simulink model "basicSISOsimulation"  (R2019b)
settings: Solver=VariableStepAuto  StartTime=0.0  StopTime=2  FixedStep=0.05  RelTol=1e-3
PreLoadFcn:
  | loadSystemVariables
values from neighbouring files (symbols this model uses):
  I = qpar('I',0.050,0.040,0.060,50)    [SISO_phi.m]    (also in SISO_x.m = 0.05; basicSISO_phi.m; basicSISO_x.m = 0.05; basicSISO_y.m = 0.05)
  m_nom = 1    [SISO_x.m]    (also in basicSISO_x.m; basicSISO_y.m; loadSystemVariables.m)
  tau = 0.075    [loadSystemVariables.m]
  tau2 = qpar('tau2',0.060,0.050,0.070,50)    [SISO_phi.m]    (also in loadSystemVariables.m = 0.06)
libraries: cstblocks x8, simulink_extras x2, aerolibguid x1, simulink x1
settings Model: Creator=Iftah  LastModifiedBy=Iftah
settings SolverCC: ZeroCrossAlgorithm=Adaptive  AlgebraicLoopSolver=LineSearch
settings DebuggingCC: IgnoredZcDiagnostic=none

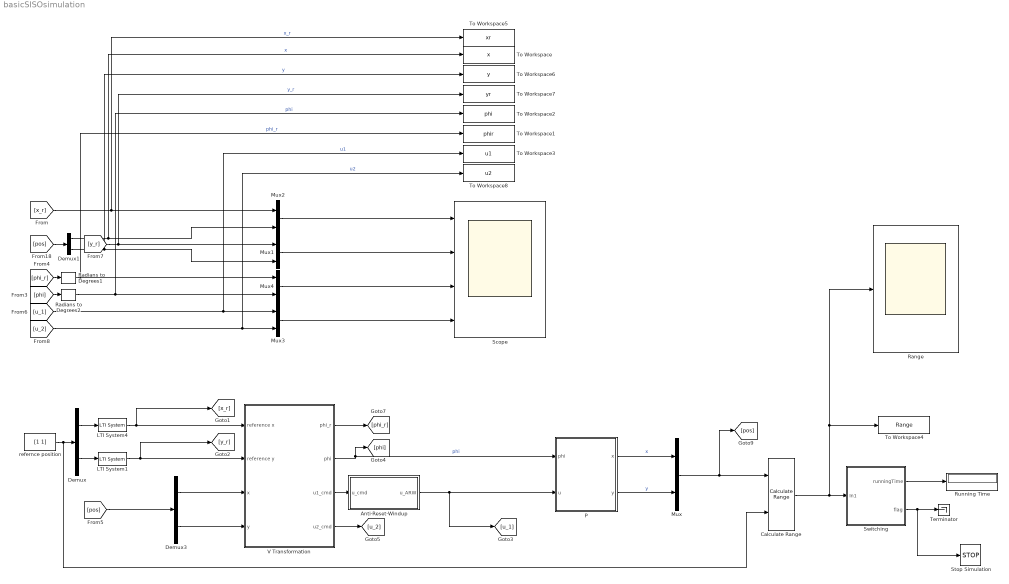
== system basicSISOsimulation ==
  Anti-Reset-Windup : Subsystem
  Calculate Range : aerolibguid/Calculate Range
      settings: SourceProductName=Aerospace Blockset  SourceProductBaseCode=AE
  Demux : Demux  Outputs=2
  Demux1 : Demux  Outputs=2
  Demux3 : Demux  Outputs=2
  LTI System1 : cstblocks/LTI System  sys=Fv  IC=[]
  LTI System4 : cstblocks/LTI System  sys=Fv  IC=[]
  Mux{,1..4} (5 alike) : Mux  Inputs=2
  P : Subsystem
  Radians to Degrees1 : simulink_extras/Transformations/Radians to Degrees
  Radians to Degrees2 : simulink_extras/Transformations/Radians to Degrees
  Range : Scope
  Running Time : Display
  Scope : Scope  NumInputPorts=4
  Stop Simulation : Stop
  Switching : Subsystem
  Terminator : Terminator
  To Workspace : ToWorkspace  VariableName=x  SaveFormat=Timeseries  SampleTime=-1
  To Workspace1 : ToWorkspace  VariableName=phir  SaveFormat=Timeseries  SampleTime=-1
  To Workspace2 : ToWorkspace  VariableName=phi  SaveFormat=Timeseries  SampleTime=-1
  To Workspace3 : ToWorkspace  VariableName=u1  SaveFormat=Timeseries  SampleTime=-1
  To Workspace4 : ToWorkspace  VariableName=Range  SaveFormat=Timeseries  SampleTime=-1
  To Workspace5 : ToWorkspace  VariableName=xr  SaveFormat=Timeseries  SampleTime=-1
  To Workspace6 : ToWorkspace  VariableName=y  SaveFormat=Timeseries  SampleTime=-1
  To Workspace7 : ToWorkspace  VariableName=yr  SaveFormat=Timeseries  SampleTime=-1
  To Workspace8 : ToWorkspace  VariableName=u2  SaveFormat=Timeseries  SampleTime=-1
  V Transformation : Subsystem
  "refernce position " : Constant  Value=[1 1]
  wires:
  "refernce position "/1 -> Demux/1, Calculate Range/2
  Demux/1 -> LTI System4/1
  Demux/2 -> LTI System1/1
  V Transformation/2(phi) -> [phi], P/1(phi)  "phi"
  Mux1/1 -> Scope/2
  Mux2/1 -> Scope/1
  [x_r] -> To Workspace5/1, Mux2/1  "x_r"
  Demux1/1 -> To Workspace/1, Mux2/2  "x"
  Demux1/2 -> Mux1/2, To Workspace6/1  "y"
  [y_r] -> Mux1/1, To Workspace7/1  "y_r"
  Mux4/1 -> Scope/3
  Mux3/1 -> Scope/4
  [u_1] -> To Workspace3/1, Mux3/1  "u1"
  [u_2] -> To Workspace8/1, Mux3/2  "u2"
  V Transformation/1(phi_r) -> [phi_r]
  [phi_r] -> Radians to Degrees1/1
  [phi] -> Radians to Degrees2/1
  Radians to Degrees1/1 -> Mux4/1, To Workspace1/1  "phi_r"
  Radians to Degrees2/1 -> To Workspace2/1, Mux4/2  "phi"
  P/1(x) -> Mux/1  "x"
  P/2(y) -> Mux/2  "y"
  Demux3/1 -> V Transformation/3(x)
  Demux3/2 -> V Transformation/4(y)
  Calculate Range/1 -> Switching/1(In1), To Workspace4/1, Range/1
  Switching/1(runningTime) -> Running Time/1
  LTI System4/1 -> [x_r], V Transformation/1(reference x)
  LTI System1/1 -> [y_r], V Transformation/2(reference y)
  [pos] -> Demux1/1
  V Transformation/4(u2_cmd) -> [u_2]
  Switching/2("flag ") -> Stop Simulation/1, Terminator/1
  Mux/1 -> [pos], Calculate Range/1
  [pos] -> Demux3/1
  V Transformation/3(u1_cmd) -> Anti-Reset-Windup/1(u_cmd)
  Anti-Reset-Windup/1(u_ARW) -> P/2("u "), [u_1]

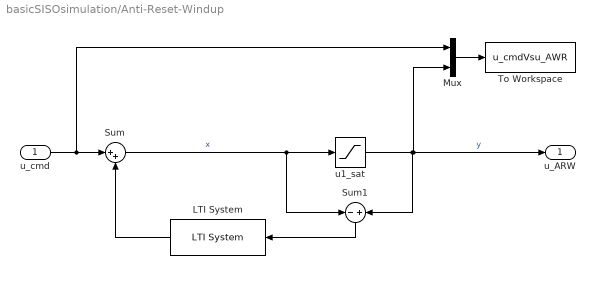
== system basicSISOsimulation/Anti-Reset-Windup ==
  u_cmd : Inport
  LTI System : cstblocks/LTI System  sys=Hv  IC=[]
  Mux : Mux  Inputs=2
  Sum : Sum  Inputs=|++
  Sum1 : Sum  Inputs=-|+
  To Workspace : ToWorkspace  VariableName=u_cmdVsu_AWR  SaveFormat=Timeseries  SampleTime=-1
  u1_sat : Saturate  UpperLimit=25  LowerLimit=-25
  u_ARW : Outport
  wires:
  u_cmd/1 -> Mux/1, Sum/1
  u1_sat/1 -> Mux/2, u_ARW/1, Sum1/2  "y"
  Sum/1 -> Sum1/1, u1_sat/1  "x"
  Sum1/1 -> LTI System/1
  LTI System/1 -> Sum/2
  Mux/1 -> To Workspace/1

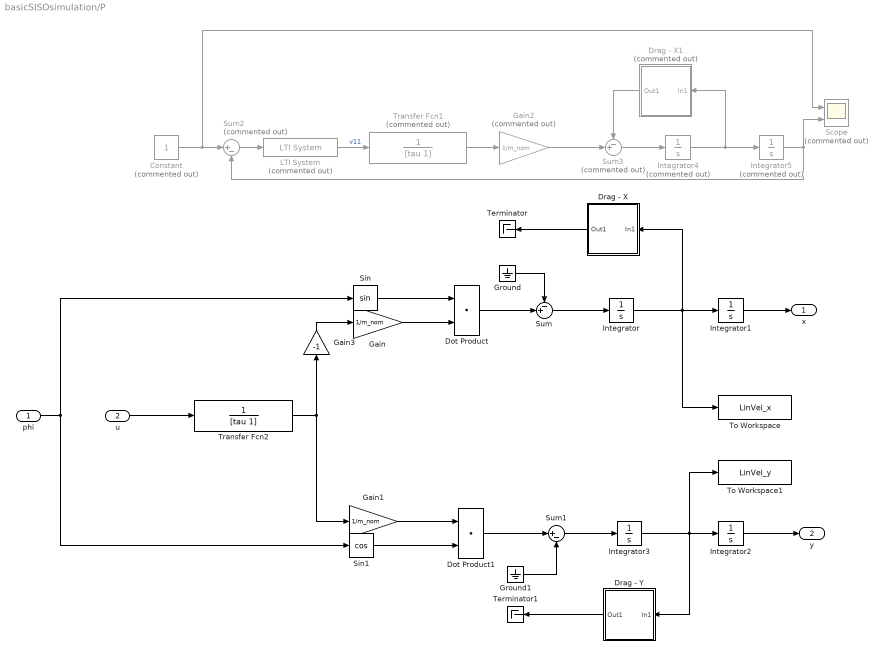
== system basicSISOsimulation/P ==
  phi : Inport
  "u " : Inport  Port=2
  Constant : Constant  Commented=on
  Dot Product : DotProduct  InputSameDT=on  OutDataTypeStr=Inherit: Inherit via internal rule
  Dot Product1 : DotProduct  InputSameDT=on  OutDataTypeStr=Inherit: Inherit via internal rule
  Drag - X : Subsystem
  Drag - X1 : Subsystem  Commented=on
  Drag - Y : Subsystem
  Gain : Gain  Gain=1/m_nom
  Gain1 : Gain  Gain=1/m_nom
  Gain2 : Gain  Commented=on  Gain=1/m_nom
  Gain3 : Gain  Gain=-1
  Ground : Ground
  Ground1 : Ground
  Integrator : Integrator
  Integrator1 : Integrator  InitialCondition=1e-3
  Integrator2 : Integrator  InitialCondition=1e-3
  Integrator3 : Integrator
  Integrator4 : Integrator  Commented=on  InitialCondition=1e-3
  Integrator5 : Integrator  Commented=on  InitialCondition=1e-3
  LTI System : cstblocks/LTI System  Commented=on  sys=Gv  IC=[]
  Scope : Scope  Commented=on  NumInputPorts=2
  Sin : Trigonometry
  Sin1 : Trigonometry  Operator=cos
  Sum : Sum  Inputs=-+|
  Sum1 : Sum  Inputs=|+-
  Sum2 : Sum  Commented=on  Inputs=|+-
  Sum3 : Sum  Commented=on  Inputs=-+|
  Terminator : Terminator
  Terminator1 : Terminator
  To Workspace : ToWorkspace  VariableName=LinVel_x  SaveFormat=Timeseries  SampleTime=-1
  To Workspace1 : ToWorkspace  VariableName=LinVel_y  SaveFormat=Timeseries  SampleTime=-1
  Transfer Fcn1 : TransferFcn  Commented=on  Denominator=[tau 1]
  Transfer Fcn2 : TransferFcn  Denominator=[tau 1]
  x : Outport
  y : Outport  Port=2
  wires:
  Gain/1 -> Dot Product/2
  Integrator1/1 -> x/1
  Integrator3/1 -> Drag - Y/1(In1), To Workspace1/1, Integrator2/1
  phi/1 -> Sin/1, Sin1/1
  Sin1/1 -> Dot Product1/2
  Gain3/1 -> Gain/1
  Gain1/1 -> Dot Product1/1
  "u "/1 -> Transfer Fcn2/1
  Transfer Fcn2/1 -> Gain1/1, Gain3/1
  Sin/1 -> Dot Product/1
  Integrator/1 -> To Workspace/1, Integrator1/1, Drag - X/1(In1)
  Sum/1 -> Integrator/1
  Sum1/1 -> Integrator3/1
  Drag - Y/1(Out1) -> Terminator1/1
  Dot Product/1 -> Sum/2
  Dot Product1/1 -> Sum1/1
  Transfer Fcn1/1 -> Gain2/1
  LTI System/1 -> Transfer Fcn1/1  "v11"
  Sum2/1 -> LTI System/1
  Constant/1 -> Scope/1, Sum2/1
  Integrator2/1 -> y/1
  Integrator4/1 -> Drag - X1/1(In1), Integrator5/1
  Gain2/1 -> Sum3/2
  Integrator5/1 -> Scope/2, Sum2/2
  Sum3/1 -> Integrator4/1
  Drag - X1/1(Out1) -> Sum3/1
  Drag - X/1(Out1) -> Terminator/1
  Ground/1 -> Sum/1
  Ground1/1 -> Sum1/2

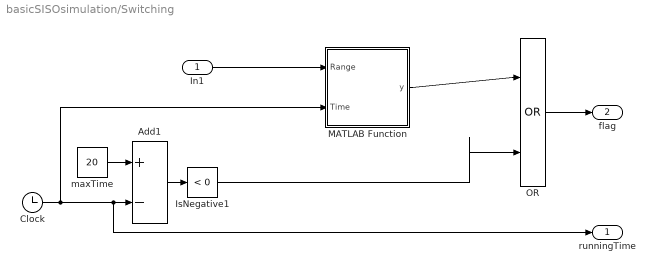
== system basicSISOsimulation/Switching ==
  In1 : Inport
  Add1 : Sum  Inputs=+-
  Clock : Clock
  IsNegative1 : simulink/Logic and Bit Operations/Compare To Zero  relop=<  OutDataTypeStr=boolean
  MATLAB Function : MATLAB Function  TreatAsAtomicUnit=on
  OR : Logic  Operator=OR  IconShape=distinctive  AllPortsSameDT=off  OutDataTypeStr=boolean
  maxTime : Constant  Value=20
  runningTime : Outport
  "flag " : Outport  Port=2
  wires:
  OR/1 -> "flag "/1
  IsNegative1/1 -> OR/2
  Add1/1 -> IsNegative1/1
  In1/1 -> MATLAB Function/1(Range)
  Clock/1 -> MATLAB Function/2(Time), runningTime/1, Add1/2
  maxTime/1 -> Add1/1
  MATLAB Function/1(y) -> OR/1

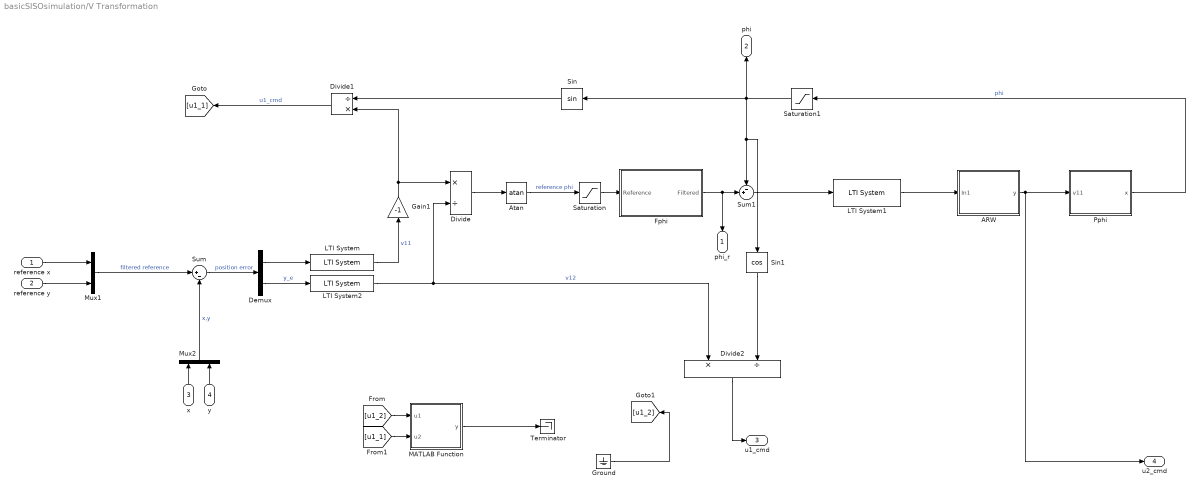
== system basicSISOsimulation/V Transformation ==
  reference x : Inport
  reference y : Inport  Port=2
  x : Inport  Port=3
  y : Inport  Port=4
  ARW : Subsystem
  Atan : Trigonometry  Operator=atan
  Demux : Demux  Outputs=2
  Divide : Product  Inputs=*/
  Divide1 : Product  Inputs=/*
  Divide2 : Product  Inputs=*/
  Fphi : Subsystem
  Gain1 : Gain  Gain=-1
  Ground : Ground
  LTI System : cstblocks/LTI System  sys=Gv  IC=[]
  LTI System1 : cstblocks/LTI System  sys=Gphi  IC=[]
  LTI System2 : cstblocks/LTI System  sys=Gv  IC=[]
  MATLAB Function : MATLAB Function  TreatAsAtomicUnit=on
  Mux1 : Mux  Inputs=2
  Mux2 : Mux  Inputs=2
  Pphi : Subsystem
  Saturation : Saturate  UpperLimit=pi/3  LowerLimit=-pi/3
  Saturation1 : Saturate  UpperLimit=pi/3  LowerLimit=-pi/3
  Sin : Trigonometry
  Sin1 : Trigonometry  Operator=cos
  Sum : Sum  Inputs=|+-
  Sum1 : Sum  Inputs=-+|
  Terminator : Terminator
  phi_r : Outport
  phi : Outport  Port=2
  u1_cmd : Outport  Port=3
  u2_cmd : Outport  Port=4
  wires:
  Divide/1 -> Atan/1
  LTI System2/1 -> Divide2/1, Divide/2  "v12"
  Pphi/1(x) -> Saturation1/1  "phi"
  Sum/1 -> Demux/1  "position error"
  Sum1/1 -> LTI System1/1
  Demux/2 -> LTI System2/1  "y_e"
  Mux1/1 -> Sum/1  "filtered reference"
  Atan/1 -> Saturation/1  "reference phi"
  y/1 -> Mux2/2
  x/1 -> Mux2/1
  Mux2/1 -> Sum/2  "x,y"
  reference y/1 -> Mux1/2
  reference x/1 -> Mux1/1
  Sin1/1 -> Divide2/2
  Gain1/1 -> Divide/1, Divide1/2
  LTI System/1 -> Gain1/1  "v11"
  Divide1/1 -> [u1_1]  "u1_cmd"
  Sin/1 -> Divide1/1
  Divide2/1 -> u1_cmd/1
  Demux/1 -> LTI System/1
  [u1_2] -> MATLAB Function/1(u1)
  [u1_1] -> MATLAB Function/2(u2)
  MATLAB Function/1(y) -> Terminator/1
  Fphi/1(Filtered) -> Sum1/2, phi_r/1
  LTI System1/1 -> ARW/1(In1)
  Ground/1 -> [u1_2]
  ARW/1(y) -> Pphi/1(v11), u2_cmd/1
  Saturation/1 -> Fphi/1(Reference)
  Saturation1/1 -> Sum1/1, Sin1/1, Sin/1, phi/1

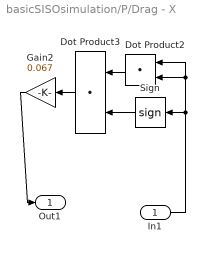
== system basicSISOsimulation/P/Drag - X ==
  In1 : Inport
  Dot Product2 : DotProduct  InputSameDT=on  OutDataTypeStr=Inherit: Inherit via internal rule
  Dot Product3 : DotProduct  InputSameDT=on  OutDataTypeStr=Inherit: Inherit via internal rule
  Gain2 : Gain  Gain=0.067
  Sign : Signum
  Out1 : Outport
  wires:
  In1/1 -> Dot Product2/1, Dot Product2/2, Sign/1
  Dot Product2/1 -> Dot Product3/1
  Sign/1 -> Dot Product3/2
  Dot Product3/1 -> Gain2/1
  Gain2/1 -> Out1/1

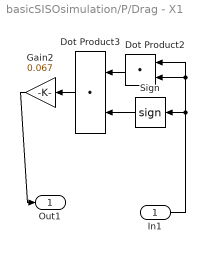
== system basicSISOsimulation/P/Drag - X1 ==
  In1 : Inport
  Dot Product2 : DotProduct  InputSameDT=on  OutDataTypeStr=Inherit: Inherit via internal rule
  Dot Product3 : DotProduct  InputSameDT=on  OutDataTypeStr=Inherit: Inherit via internal rule
  Gain2 : Gain  Gain=0.067
  Sign : Signum
  Out1 : Outport
  wires:
  Gain2/1 -> Out1/1
  Dot Product3/1 -> Gain2/1
  Sign/1 -> Dot Product3/2
  Dot Product2/1 -> Dot Product3/1
  In1/1 -> Sign/1, Dot Product2/2, Dot Product2/1

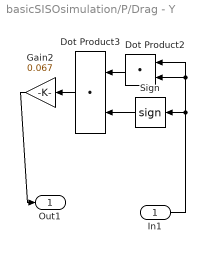
== system basicSISOsimulation/P/Drag - Y ==
  In1 : Inport
  Dot Product2 : DotProduct  InputSameDT=on  OutDataTypeStr=Inherit: Inherit via internal rule
  Dot Product3 : DotProduct  InputSameDT=on  OutDataTypeStr=Inherit: Inherit via internal rule
  Gain2 : Gain  Gain=0.067
  Sign : Signum
  Out1 : Outport
  wires:
  Gain2/1 -> Out1/1
  Dot Product3/1 -> Gain2/1
  Sign/1 -> Dot Product3/2
  Dot Product2/1 -> Dot Product3/1
  In1/1 -> Sign/1, Dot Product2/2, Dot Product2/1

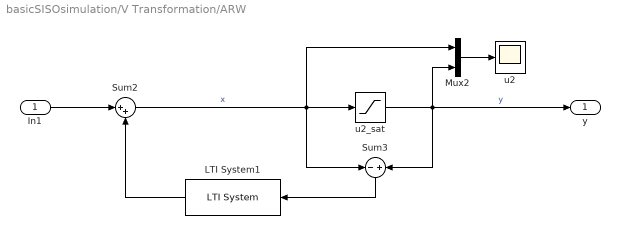
== system basicSISOsimulation/V Transformation/ARW ==
  In1 : Inport
  LTI System1 : cstblocks/LTI System  sys=Hphi  IC=[]
  Mux2 : Mux  Inputs=2
  Sum2 : Sum  Inputs=|++
  Sum3 : Sum  Inputs=-|+
  u2 : Scope
  u2_sat : Saturate  UpperLimit=10  LowerLimit=-10
  y : Outport
  wires:
  In1/1 -> Sum2/1
  Sum3/1 -> LTI System1/1
  Mux2/1 -> u2/1
  u2_sat/1 -> Sum3/2, Mux2/2, y/1  "y"
  Sum2/1 -> Sum3/1, Mux2/1, u2_sat/1  "x"
  LTI System1/1 -> Sum2/2

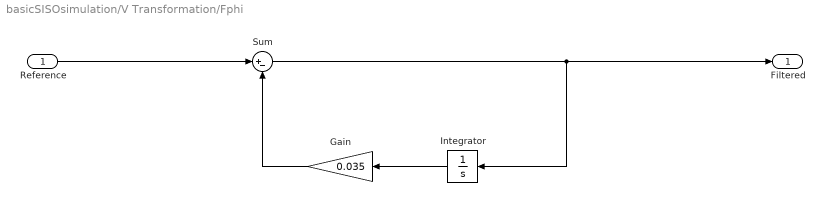
== system basicSISOsimulation/V Transformation/Fphi ==
  Reference : Inport
  Gain : Gain  Gain=0.035
  Integrator : Integrator  InitialCondition=pi/100  LowerSaturationLimit=-1000
  Sum : Sum  Inputs=|+-
  Filtered : Outport
  wires:
  Reference/1 -> Sum/1
  Sum/1 -> Integrator/1, Filtered/1
  Integrator/1 -> Gain/1
  Gain/1 -> Sum/2

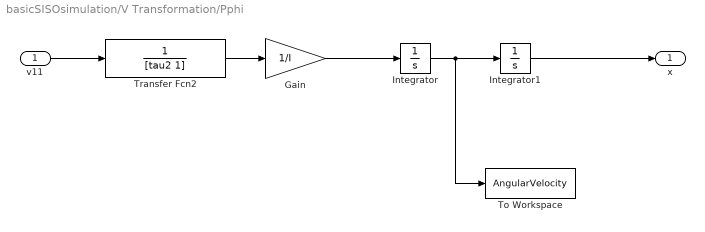
== system basicSISOsimulation/V Transformation/Pphi ==
  v11 : Inport
  Gain : Gain  Gain=1/I
  Integrator : Integrator
  Integrator1 : Integrator  InitialCondition=-pi/4
  To Workspace : ToWorkspace  VariableName=AngularVelocity  SaveFormat=Timeseries  SampleTime=-1
  Transfer Fcn2 : TransferFcn  Denominator=[tau2 1]
  x : Outport
  wires:
  Gain/1 -> Integrator/1
  Integrator/1 -> To Workspace/1, Integrator1/1
  v11/1 -> Transfer Fcn2/1
  Integrator1/1 -> x/1
  Transfer Fcn2/1 -> Gain/1

== matlab function basicSISOsimulation/V Transformation/MATLAB Function ==
  data: u1 input; y output; u2 input
function y = fcn(u1,u2)
y = ((abs(u1)+abs(u2))/2) * sign(u1);

== matlab function basicSISOsimulation/Switching/MATLAB Function ==
  settings: updateMethod=DISCRETE
  data: Range input; y output; Time input
function y = fcn(Range,Time)
persistent oldRange

if isempty(oldRange)
    oldRange = Range * 2;
end

if Time < 0.1
    y = 0;
else
    if Range < oldRange
        y = 0;
    else
        y = 1;
    end
end
oldRange = Range;
